simulink model "bodymodel"  (R2018b)
settings: Solver=VariableStepAuto  StartTime=0.0  StopTime=10.0  RelTol=1e-3
values from neighbouring files (symbols this model uses):
  cs = 1000    [baseVehicleData.mat]    (also in initModel.m)
  ks = 20000    [baseVehicleData.mat]    (also in initModel.m; initModelQuarter.m)
  m = 250    [baseVehicleData.mat]
settings Model: Creator=Jamie  LastModifiedBy=Jamie

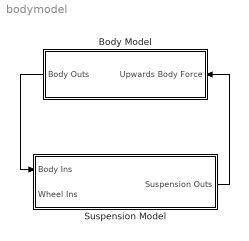
== system bodymodel ==
  Body Model : Subsystem
  Suspension Model : Subsystem
  wires:
  Body Model/1(Body Outs) -> Suspension Model/1(Body Ins)
  Suspension Model/1(Suspension Outs) -> Body Model/1(Upwards Body Force)

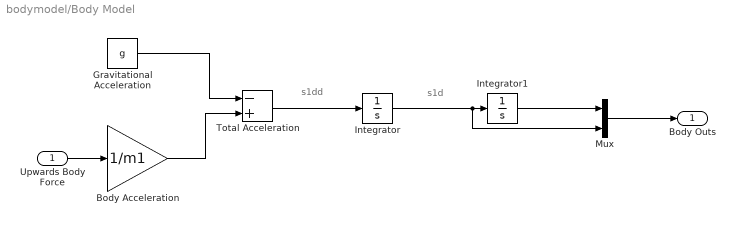
== system bodymodel/Body Model ==
  note: s1d
  note: s1dd
  Upwards Body Force : Inport
  Body Acceleration : Gain  Gain=1/m1  mask{m1=500}
      mask prompts: m1 "Body Mass"
  Gravitational Acceleration : Constant  Value=g  mask{g=9.81}
      mask prompts: g "Gravitational Acceleration"
  Integrator : Integrator
  Integrator1 : Integrator
  Mux : Mux  Inputs=2
  Total Acceleration : Sum  Inputs=-+
  Body Outs : Outport
  wires:
  Integrator1/1 -> Mux/1
  Total Acceleration/1 -> Integrator/1
  Body Acceleration/1 -> Total Acceleration/2
  Integrator/1 -> Mux/2, Integrator1/1
  Mux/1 -> Body Outs/1
  Gravitational Acceleration/1 -> Total Acceleration/1
  Upwards Body Force/1 -> Body Acceleration/1

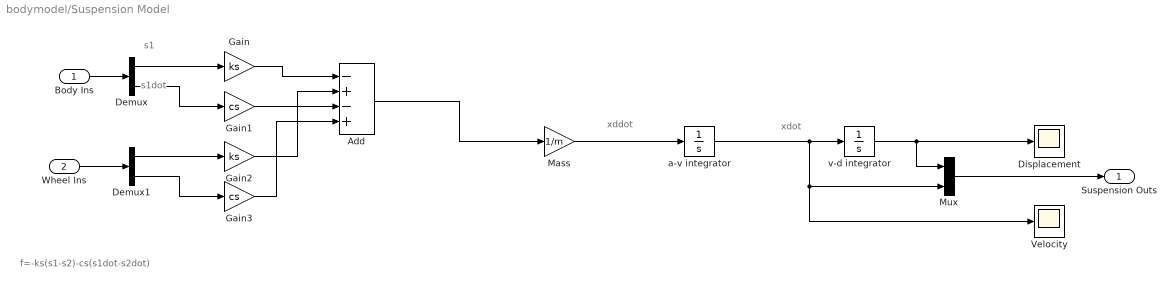
== system bodymodel/Suspension Model ==
  note: f=-ks(s1-s2)-cs(s1dot-s2dot)
  note: s1dot
  note: s1
  note: xdot
  note: xddot
  Body Ins : Inport
  Wheel Ins : Inport  Port=2
  Add : Sum  Inputs=-+-+
  Demux : Demux  Outputs=2
  Demux1 : Demux  Outputs=2
  Displacement : Scope
  Gain : Gain  Gain=ks
  Gain1 : Gain  Gain=cs
  Gain2 : Gain  Gain=ks
  Gain3 : Gain  Gain=cs
  Mass : Gain  Gain=1/m
  Mux : Mux  Inputs=2
  Velocity : Scope
  a-v integrator : Integrator
  v-d integrator : Integrator
  Suspension Outs : Outport
  wires:
  v-d integrator/1 -> Displacement/1, Mux/1
  Mass/1 -> a-v integrator/1
  Body Ins/1 -> Demux/1
  Demux/1 -> Gain/1
  Demux/2 -> Gain1/1
  Gain/1 -> Add/1
  Gain1/1 -> Add/3
  Add/1 -> Mass/1
  Wheel Ins/1 -> Demux1/1
  Demux1/2 -> Gain3/1
  Demux1/1 -> Gain2/1
  Gain2/1 -> Add/2
  Gain3/1 -> Add/4
  a-v integrator/1 -> Mux/2, Velocity/1, v-d integrator/1
  Mux/1 -> Suspension Outs/1
